simulink model "temp"  (R2024b)
settings: Solver=VariableStepAuto  StartTime=0.0  StopTime=10.0  RelTol=1e-3
undefined symbols (not defined in the file or in its folder): kd, ki, kp
libraries: read_b x6, send_b x5
settings Model: Creator=eikel  LastModifiedBy=eikel

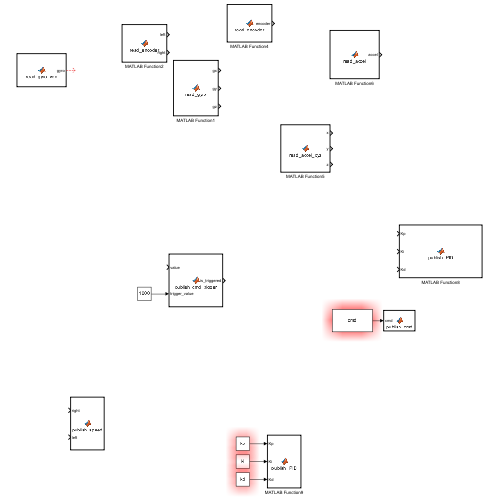
[thumbnail: Simulink's stored preview of the top-level diagram]
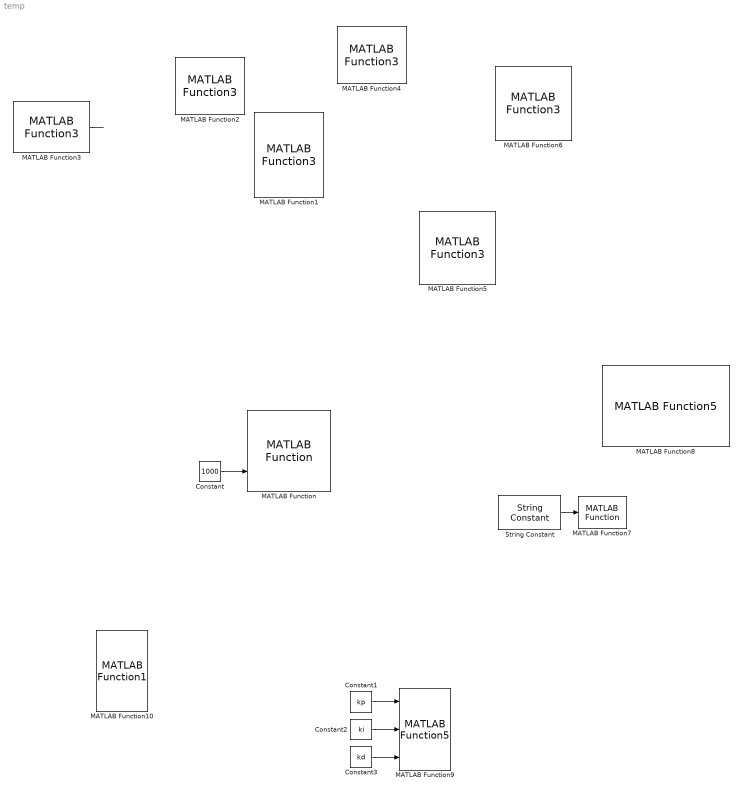
== system temp ==
  Constant : Constant  Value=1000
  Constant1 : Constant  Value=kp
  Constant2 : Constant  Value=ki
  Constant3 : Constant  Value=kd
  MATLAB Function : send_b/send command w// trigger/MATLAB Function  SystemSampleTime=-1  VariantActivationTime=update diagram  AllowFlexibleInterface=on  Latency=0  AutoFrameSizeCalculation=off
  MATLAB Function1 : read_b/read_gyro/MATLAB Function3  SystemSampleTime=-1  VariantActivationTime=update diagram  AllowFlexibleInterface=on  Latency=0  AutoFrameSizeCalculation=off
  MATLAB Function10 : send_b/send_speed_knobs/MATLAB Function1  SystemSampleTime=-1  VariantActivationTime=update diagram  AllowFlexibleInterface=on  Latency=0  AutoFrameSizeCalculation=off
  MATLAB Function2 : read_b/Subsystem2/MATLAB Function3  SystemSampleTime=-1  VariantActivationTime=update diagram  AllowFlexibleInterface=on  Latency=0  AutoFrameSizeCalculation=off
  MATLAB Function3 : read_b/read_gyro_array/MATLAB Function3  SystemSampleTime=-1  VariantActivationTime=update diagram  AllowFlexibleInterface=on  Latency=0  AutoFrameSizeCalculation=off
  MATLAB Function4 : read_b/read_encoder_array/MATLAB Function3  SystemSampleTime=-1  VariantActivationTime=update diagram  AllowFlexibleInterface=on  Latency=0  AutoFrameSizeCalculation=off
  MATLAB Function5 : read_b/read_accel/MATLAB Function3  SystemSampleTime=-1  VariantActivationTime=update diagram  AllowFlexibleInterface=on  Latency=0  AutoFrameSizeCalculation=off
  MATLAB Function6 : read_b/Subsystem1/MATLAB Function3  SystemSampleTime=-1  VariantActivationTime=update diagram  AllowFlexibleInterface=on  Latency=0  AutoFrameSizeCalculation=off
  MATLAB Function7 : send_b/send command/MATLAB Function  SystemSampleTime=-1  VariantActivationTime=update diagram  AllowFlexibleInterface=on  Latency=0  AutoFrameSizeCalculation=off
  MATLAB Function8 : send_b/Subsystem1/MATLAB Function5  SystemSampleTime=-1  VariantActivationTime=update diagram  AllowFlexibleInterface=on  Latency=0  AutoFrameSizeCalculation=off
  MATLAB Function9 : send_b/Subsystem/MATLAB Function5  SystemSampleTime=-1  VariantActivationTime=update diagram  AllowFlexibleInterface=on  Latency=0  AutoFrameSizeCalculation=off
  String Constant : StringConstant  String=cmd
  wires:
  MATLAB Function3/1 -> ?
  Constant/1 -> MATLAB Function/2
  String Constant/1 -> MATLAB Function7/1
  Constant2/1 -> MATLAB Function9/2
  Constant1/1 -> MATLAB Function9/1
  Constant3/1 -> MATLAB Function9/3
